simulink model "formation_control_old"  (R2021a)
settings: Solver=VariableStepAuto  StartTime=0.0  StopTime=T  RelTol=1e-3
undefined symbols (not defined in the file or in its folder): params
settings Model: Creator=gaeta  LastModifiedBy=giuse
settings SolverCC: AlgebraicLoopSolver=TrustRegion
settings DataIOCC: InitialState=initialCondition  LoadInitialState=on
settings DebuggingCC: SFMachineParentedDataDiag=warning

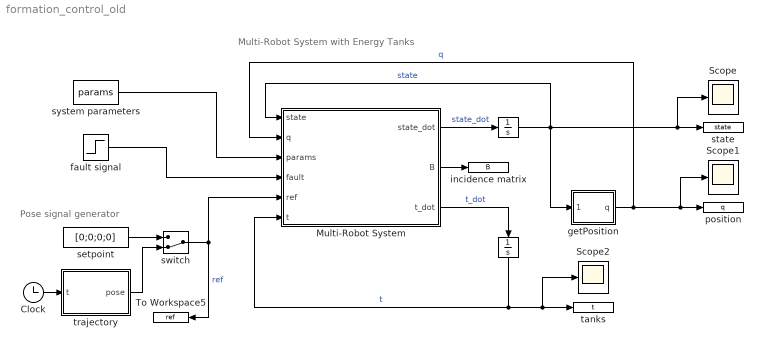
== system formation_control_old ==
  note: Multi-Robot System with Energy Tanks
  note: Pose signal generator
  "  " : Integrator
  "   " : Integrator
  Clock : Clock
  Multi-Robot System : MATLAB Function  TreatAsAtomicUnit=on
  Scope : Scope
  Scope1 : Scope
  Scope2 : Scope
  To Workspace5 : ToWorkspace  VariableName=ref  SaveFormat=Timeseries  SampleTime=-1
  fault signal : Step  Time=25  SampleTime=0
  getPosition : Subsystem
  incidence matrix : ToWorkspace  VariableName=B  SaveFormat=Timeseries  SampleTime=-1
  position : ToWorkspace  VariableName=q  SaveFormat=Timeseries  SampleTime=-1
  setpoint : Constant  Value=[0;0;0;0]
  state : ToWorkspace  VariableName=state  SaveFormat=Timeseries  SampleTime=-1
  switch : ManualSwitch  CurrentSetting=0
  "system parameters " : Constant  Value=params  OutDataTypeStr=Bus: params_bus
  tanks : ToWorkspace  VariableName=t  SaveFormat=Timeseries  SampleTime=-1
  trajectory : MATLAB Function  TreatAsAtomicUnit=on
  wires:
  trajectory/1(pose) -> switch/2
  setpoint/1 -> switch/1
  Clock/1 -> trajectory/1(t)
  switch/1 -> Multi-Robot System/5(ref), To Workspace5/1  "ref"
  "system parameters "/1 -> Multi-Robot System/3(params)
  fault signal/1 -> Multi-Robot System/4(fault)
  "  "/1 -> Multi-Robot System/6(t), tanks/1, Scope2/1  "t"
  Multi-Robot System/1(state_dot) -> "   "/1  "state_dot"
  Multi-Robot System/2(B) -> incidence matrix/1
  "   "/1 -> Multi-Robot System/1(state), Scope/1, state/1, getPosition/1(state)  "state"
  Multi-Robot System/3(t_dot) -> "  "/1  "t_dot"
  getPosition/1(q) -> Scope1/1, position/1, Multi-Robot System/2(q)  "q"

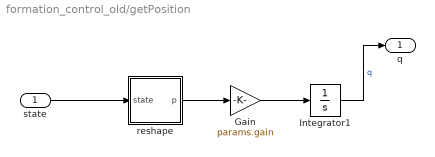
== system formation_control_old/getPosition ==
  state : Inport
  Gain : Gain  Gain=params.gain
  Integrator1 : Integrator
  reshape : MATLAB Function  TreatAsAtomicUnit=on
  q : Outport
  wires:
  state/1 -> reshape/1(state)
  reshape/1(p) -> Gain/1
  Gain/1 -> Integrator1/1
  Integrator1/1 -> q/1  "q"

== matlab function formation_control_old/trajectory ==
  data: pose output size=4; t input size=1
%% generate reference trajectory
function pose = trajectory(t)
t1 = 5;
t_fault = 25;
t_end = 55;
pause = 5;

w = 0.25;
phi = -w*t1;
A = 80;
z_vel = 1;

y = [0;0;0];
theta = pi/2;
if(t>=t1 && t<t_fault)
    y = [A*sin(w*t+phi); -A*cos(w*t+phi); z_vel*t] - [A*sin(w*t1+phi); -A*cos(w*t1+phi); z_vel*t1];
    theta = atan2(A*sin(w*t+phi), A*cos(w*t+phi));
elseif(t>=t_fault && t<t_fault+pause)
    y = [A*sin(w*t_fault+phi); -A*cos(w*t_fault+phi); z_vel*t_fault] - [A*sin(w*t1+phi); -A*cos(w*t1+phi); z_vel*t1];
    theta = atan2(A*sin(w*t_fault+phi), A*cos(w*t_fault+phi));
elseif(t>=t_fault+pause && t<t_end)
    y = [A*sin(w*(t-pause)+phi); -A*cos(w*(t-pause)+phi); z_vel*(t-pause)] - [A*sin(w*t1+phi); -A*cos(w*t1+phi); z_vel*t1];
    theta = atan2(A*sin(w*(t-pause)+phi), A*cos(w*(t-pause)+phi));
elseif(t>=t_end)
    y = [A*sin(w*(t_end-pause)+phi); -A*cos(w*(t_end-pause)+phi); z_vel*(t_end-pause)] - [A*sin(w*t1+phi); -A*cos(w*t1+phi); z_vel*t1];
    theta = atan2(A*sin(w*(t_end-pause)+phi), A*cos(w*(t_end-pause)+phi));
end

pose = [y; theta];
end

== matlab function formation_control_old/Multi-Robot System ==
  data: state input size=3*(params.N+params.E); q input size=3*params.N; state_dot output size=3*(params.N+params.E); params input; fault input; ref input size=4; t input size=params.N; B output; t_dot output size=params.N
function [state_dot,B,t_dot] = closedLoopSystem(state, q, params, fault, ref, t)
n = 3;                      % task space
N = params.N;               % number of robots
faulted_robot = params.faulted_robot;

%% initialize some matrices
p = state(1:n*N);           % robots momenta
m = params.m;               % robots masses
M = zeros(n*N, n*N);      	% inertia matrix
d = params.d;               % frict. coeff
D = zeros(n*N, n*N);        % system dissipation matrix
for i = 1:N
    M(n*i-n+1:n*i, n*i-n+1:n*i) = eye(n).*m(i);
    D(n*i-n+1:n*i, n*i-n+1:n*i) = eye(n).*d(i);
end

E = params.E;               % number of edges

%% Check whether a fault is occurred
joined_e = 0;
if(sum(fault)~=0 && ~params.fault_occurred)
    params.fault_occurred = 1;  % flag on
    [params.B, joined_e] = faultHandler(params.B, params.Bfull, faulted_robot);
end

%% Still initialize matrices
B = params.B;
Bcl = kron(params.B,eye(n));	% closed-loop incidence matrix

dc = params.dc;             % robots dissipations
Dc = zeros(n*E, n*E);       % controller dissipation matrix
kc = params.kc;             % constant springs
Kc = zeros(n*E, n*E);       % constant spring matrix
R = zeros(n*E, n*E);        % n*E matrix containing E rotation matrices

for j = 1:E
    Dc(n*j-n+1:n*j, n*j-n+1:n*j) = eye(n).*dc(j);
    Kc(n*j-n+1:n*j, n*j-n+1:n*j) = eye(n).*kc(j);
    R(n*j-n+1:n*j, n*j-n+1:n*j) = rotz(ref(4)-pi/2);
end

z = state(n*N+1:n*(N+E));	% edges lengths
z_des = R*params.z_des;     % desired edges lengths

% NOTE: constant matrices M, D, Dc, Kc should be moved in the Init file

%% Energy transfer protocol
t_dot = zeros(size(t));     % tanks dynamics
w = zeros(E*n,1);           % additional input for energy transfer

if(params.fault_occurred) 
    Fa_ij = zeros(n,1);
    for i = 1:n
        Fa_ij(i) = Vdot( z(joined_e*n-n+i)-z_des(joined_e*n-n+i) );
    end
    
    i = find(B(:,joined_e)==-1);
    j = find(B(:,joined_e)==1);
    
    Diss = p.'*(inv(M).'*D*inv(M))*p;       % energy dissipation
    
    %update tank i
    wt_ij = -params.gamma(joined_e)*(Fa_ij.'*Fa_ij)*t(i);
    t_dot_i = Diss/t(i) + wt_ij;
    if( all(t(i)>params.tank_max & t_dot_i>0) || all(t(i)<params.tank_min & t_dot_i<0) )
        t_dot(i) = 0;
    else
        t_dot(i) = t_dot_i;
    end
    
    %update tank j
    wt_ji = -params.gamma(joined_e)*(Fa_ij.'*Fa_ij)*t(j);
    t_dot_j = Diss/t(j) + wt_ji;
    if( all(t(j)>params.tank_max & t_dot_j>0) || all(t(j)<params.tank_min & t_dot_j<0) )
        t_dot(j) = 0;
    else
        t_dot(j) = t_dot_j;
    end
    
    % update w
    wz_ij = -params.gamma(joined_e)*Fa_ij*t(i)^2 - params.gamma(joined_e)*Fa_ij*t(j)^2;
    w(joined_e*n-n+1:joined_e*n) = wz_ij;
end

%% Trajectory Tracking / Setpoint Regulation
tracking = true;    % #CHANGE THIS: ENABLE/DISABLE TRAJECTORY TRACKING
u = zeros(n*N,1);
if(tracking)
    
    % control for leader trajectory tracking
    Kp = 20;
    u(1:n) = Kp*(ref(1:n)-q(1:n));
    
    % control for faulted robot
    K_pd = 0.4;
    P_action = K_pd*(1-q(n*faulted_robot));
	D_action = K_pd*p(n*faulted_robot)/m(faulted_robot);
    u(n*faulted_robot) = params.fault_occurred*(P_action-D_action);
end

%% Multi-robot System Dynamics
Fe = -Bcl * Kc*(z-z_des);           % external forces (control action)
Fa = -(Bcl*Dc*Bcl.')*(M^(-1)*p);    % interaction (coupling) forces
p_dot = Fa + Fe - D*(M^(-1)*p) + u;
z_dot = Bcl.'*(M^(-1)*p) + w;
state_dot = [p_dot; z_dot];

end


%% Potential energy function ----------------------------------------------
function v = V(error)
if (error<=0)
    v = error^2;
elseif(error>=0 && error<5*pi)
    v = 50*cos(0.2*error-pi)+50;
else
    v = 100;
end
end

%% Derivative of the Potential energy function
function vdot = Vdot(error)
if (error<=0)
    vdot = 2*error;
elseif(error>0 && error<5*pi)
    vdot = 10*sin(0.2*error);
else
    vdot = 0;
end
end

%% Split & Join operations
function [B, joined_edge] = faultHandler(B, Bfull, faulted_robot)
% split
if(faulted_robot==1)
    disp("leader cannot be faulted by hypothesis");
else
    faulted_edges = getEdges(faulted_robot, B);
    for e = 1:size(B,2)
        if(ismember(e,faulted_edges))
           B(:,e) = zeros(size(B,1),1); 
        end
    end
end

% join
if(faulted_robot==size(B,1))
    i = faulted_robot-1;
    j = 1;
else
    i = faulted_robot-1;
    j = faulted_robot+1;
end
joined_edge = getEdge(i,j,Bfull);
B(:,joined_edge) = Bfull(:,joined_edge);
end

% given a robot, return connected edges
function edges = getEdges(robot, B)
edges = find(B(robot,:)~=0);
end

% given 2 robots, return the edge connecting them, 0 otherwise
function edge = getEdge(i, j, B)
edge = 0;
for e = 1:size(B,2)
    if( (B(i,e)==1 && B(j,e)==-1) || (B(i,e)==-1 && B(j,e)==1) )
        edge = e;
        break
    end
end
end

%

== matlab function formation_control_old/getPosition/reshape ==
  data: p output size=3*params.N; state input size=3*(params.N+params.E)
function p = reshape(state)
    %n = 3;
    %N = roots([n/2, n/2, -size(state,1)]).'*(roots([n/2, n/2, -size(state,1)])>0);
    N = 5;
    p = state(1:3*5);
end




%
